simulink model "pmsm_hil"  (R2018b)
settings: Solver=VariableStepAuto  StartTime=0.0  StopTime=10.0  RelTol=1e-3
InitFcn:
  | pmsm_init;
values from neighbouring files (symbols this model uses):
  dt = 50e-9    (= 5e-08)    [pmsm_init.m]
  ImaxFX = 600    [pmsm_init.m]
  J = Tst*Tau/W    (= 0.15)    [pmsm_init.m]
  L = Ld    [pmsm_control_init.m]    (also in pmsm_init.m = [Ld Lq])
  pp = 3    [pmsm_init.m]
  Psi_PM = 66e-3    (= 0.066)    [pmsm_init.m]
  PsimaxFX = 2*abs(Psi_PM + Ld*Imax + j*Lq*Imax)    [pmsm_init.m]
  R = 18e-3    (= 0.018)    [pmsm_init.m]
  RPMmax = 60*1500/2/pi    (= 14323.9448783)    [pmsm_init.m]
  TaumaxFX = (3/2)*pp*real(j*(Psi_PM + Ld*Imax + j*Lq*Imax)*Imax*(-1+j))    [pmsm_init.m]
  Udc = 300    [pmsm_init.m]
  UmaxFX = 600    [pmsm_init.m]
  WmaxFX = 1500*pp    (= 4500)    [pmsm_init.m]
undefined symbols (not defined in the file or in its folder): j
libraries: simulink x2
settings Model: Creator=natlo  LastModifiedBy=Marci

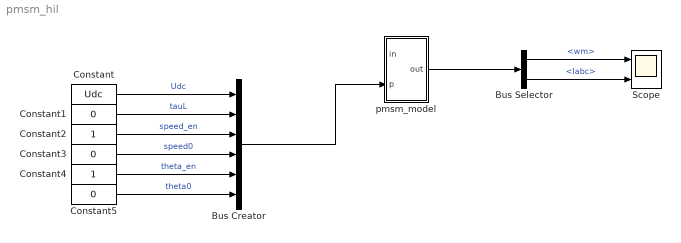
== system pmsm_hil ==
  Bus Creator : BusCreator  Inputs=6
  Bus Selector : BusSelector  OutputSignals=wm,Iabc
  Constant : Constant  Value=Udc  OutMax=[UmaxFX]  OutDataTypeStr=fixdt(1,vbits)  SampleTime=dt
  Constant1 : Constant  Value=0  OutMax=[TaumaxFX]  OutDataTypeStr=fixdt(1,vbits)  SampleTime=-1
  Constant2 : Constant  OutDataTypeStr=boolean  SampleTime=-1
  Constant3 : Constant  Value=0  OutMax=[RPMmax]  OutDataTypeStr=fixdt(1,vbits)  SampleTime=-1
  Constant4 : Constant  OutDataTypeStr=boolean  SampleTime=-1
  Constant5 : Constant  Value=0  OutMax=[180]  OutDataTypeStr=fixdt(1,vbits)  SampleTime=-1
  Scope : Scope  NumInputPorts=2
  pmsm_model : Subsystem
  wires:
  Constant5/1 -> Bus Creator/6  "theta0"
  Constant1/1 -> Bus Creator/2  "tauL"
  Constant2/1 -> Bus Creator/3  "speed_en"
  Constant/1 -> Bus Creator/1  "Udc"
  Constant3/1 -> Bus Creator/4  "speed0"
  Constant4/1 -> Bus Creator/5  "theta_en"
  Bus Creator/1 -> pmsm_model/2(p)
  pmsm_model/1(out) -> Bus Selector/1
  Bus Selector/1 -> Scope/1  "<wm>"
  Bus Selector/2 -> Scope/2  "<Iabc>"

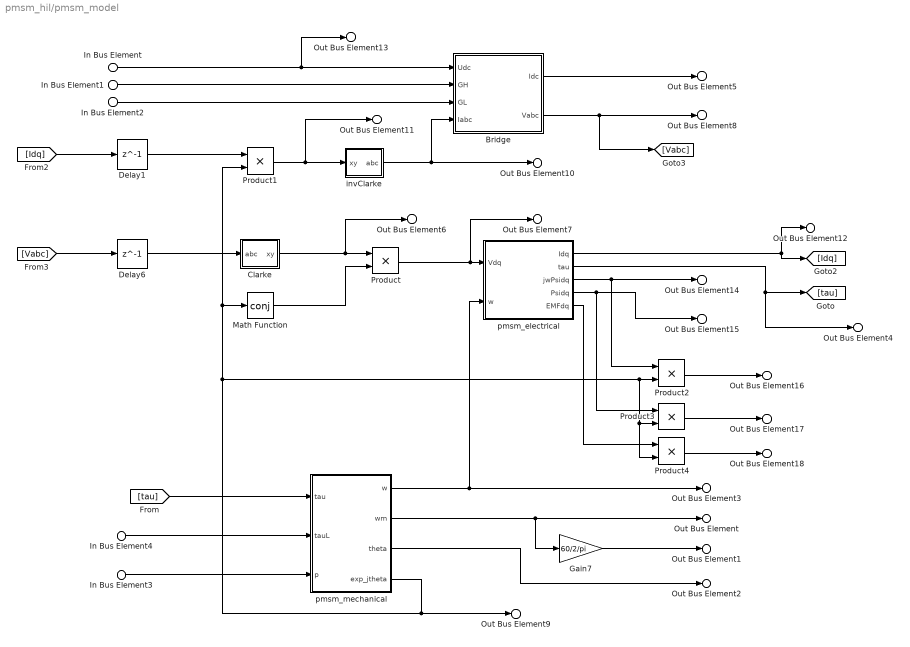
== system pmsm_hil/pmsm_model ==
  In Bus Element1 : Inport  PortName=in  Element=GH
  In Bus Element2 : Inport  PortName=in  Element=GL
  In Bus Element3 : Inport  Port=2  PortName=p
  In Bus Element : Inport  Port=2  PortName=p  Element=Udc
  In Bus Element4 : Inport  Port=2  PortName=p  Element=tauL
  Bridge : Subsystem
  Clarke : Subsystem
  Delay1 : Delay  DelayLength=1  InitialCondition=0
  Delay6 : Delay  DelayLength=1  InitialCondition=0
  Gain7 : Gain  Gain=60/2/pi  OutMax=[WmaxFX/pp*60/2/pi]  OutDataTypeStr=fixdt(1,vbits)
  Math Function : Math  Operator=conj  SaturateOnIntegerOverflow=on
  Product{,1..4} (5 alike) : Product  OutDataTypeStr=Inherit: Same as first input
  invClarke : Subsystem
  pmsm_electrical : Subsystem
  pmsm_mechanical : Subsystem
  Out Bus Element : Outport  PortName=out  Element=wm
  Out Bus Element1 : Outport  PortName=out  Element=rpm
  Out Bus Element2 : Outport  PortName=out  Element=theta
  Out Bus Element3 : Outport  PortName=out  Element=w
  Out Bus Element4 : Outport  PortName=out  Element=tau
  Out Bus Element5 : Outport  PortName=out  Element=Idc
  Out Bus Element6 : Outport  PortName=out  Element=Vxy
  Out Bus Element7 : Outport  PortName=out  Element=Vdq
  Out Bus Element8 : Outport  PortName=out  Element=Vabc
  Out Bus Element9 : Outport  PortName=out  Element=exp_jtheta
  Out Bus Element10 : Outport  PortName=out  Element=Iabc
  Out Bus Element11 : Outport  PortName=out  Element=Ixy
  Out Bus Element12 : Outport  PortName=out  Element=Idq
  Out Bus Element13 : Outport  PortName=out  Element=Udc
  Out Bus Element14 : Outport  PortName=out  Element=jwPsidq
  Out Bus Element15 : Outport  PortName=out  Element=Psidq
  Out Bus Element16 : Outport  PortName=out  Element=jwPsixy
  Out Bus Element17 : Outport  PortName=out  Element=Psixy
  Out Bus Element18 : Outport  PortName=out  Element=EMFxy
  wires:
  Product4/1 -> Out Bus Element18/1
  pmsm_electrical/5(EMFdq) -> Product4/1
  Product3/1 -> Out Bus Element17/1
  Product2/1 -> Out Bus Element16/1
  pmsm_electrical/4(Psidq) -> Product3/1, Out Bus Element15/1
  pmsm_electrical/3(jwPsidq) -> Out Bus Element14/1, Product2/1
  Delay6/1 -> Clarke/1(abc)
  Delay1/1 -> Product1/1
  In Bus Element/1 -> Bridge/1(Udc), Out Bus Element13/1
  In Bus Element1/1 -> Bridge/2(GH)
  In Bus Element2/1 -> Bridge/3(GL)
  Gain7/1 -> Out Bus Element1/1
  pmsm_mechanical/2(wm) -> Out Bus Element/1, Gain7/1
  pmsm_mechanical/3(theta) -> Out Bus Element2/1
  In Bus Element3/1 -> pmsm_mechanical/3(p)
  In Bus Element4/1 -> pmsm_mechanical/2(tauL)
  pmsm_electrical/2(tau) -> Out Bus Element4/1, [tau]
  [tau] -> pmsm_mechanical/1(tau)
  Bridge/1(Idc) -> Out Bus Element5/1
  Clarke/1(xy) -> Out Bus Element6/1, Product/1
  Math Function/1 -> Product/2
  Bridge/2(Vabc) -> Out Bus Element8/1, [Vabc]
  pmsm_mechanical/4(exp_jtheta) -> Product1/2, Math Function/1, Product2/2, Product3/2, Product4/2, Out Bus Element9/1
  [Idq] -> Delay1/1
  pmsm_electrical/1(Idq) -> Out Bus Element12/1, [Idq]
  Product/1 -> Out Bus Element7/1, pmsm_electrical/1(Vdq)
  pmsm_mechanical/1(w) -> Out Bus Element3/1, pmsm_electrical/2(w)
  [Vabc] -> Delay6/1
  Product1/1 -> invClarke/1(xy), Out Bus Element11/1
  invClarke/1(abc) -> Out Bus Element10/1, Bridge/4(Iabc)

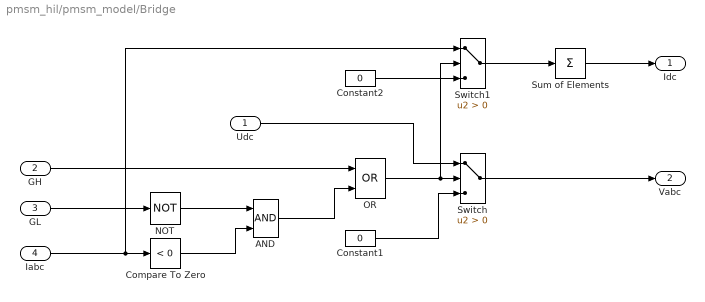
== system pmsm_hil/pmsm_model/Bridge ==
  Udc : Inport
  GH : Inport  Port=2
  GL : Inport  Port=3
  Iabc : Inport  Port=4
  AND : Logic  IconShape=distinctive  AllPortsSameDT=off  OutDataTypeStr=boolean
  Compare To Zero : simulink/Logic and Bit Operations/Compare To Zero  relop=<  OutDataTypeStr=boolean
  Constant1 : Constant  Value=0  OutDataTypeStr=Inherit: Inherit via back propagation  SampleTime=-1
  Constant2 : Constant  Value=0  OutDataTypeStr=Inherit: Inherit via back propagation  SampleTime=-1
  NOT : Logic  Operator=NOT  IconShape=distinctive  AllPortsSameDT=off  OutDataTypeStr=boolean
  OR : Logic  Operator=OR  IconShape=distinctive  AllPortsSameDT=off  OutDataTypeStr=boolean
  Sum of Elements : Sum  Inputs=+  OutMax=[ImaxFX]  OutDataTypeStr=fixdt(1,vbits)
  Switch : Switch  Criteria=u2 > Threshold
  Switch1 : Switch  Criteria=u2 > Threshold
  Idc : Outport
  Vabc : Outport  Port=2
  wires:
  Constant2/1 -> Switch1/3
  OR/1 -> Switch/2, Switch1/2
  Compare To Zero/1 -> AND/2
  Constant1/1 -> Switch/3
  GL/1 -> NOT/1
  Iabc/1 -> Switch1/1, Compare To Zero/1
  AND/1 -> OR/2
  Sum of Elements/1 -> Idc/1
  NOT/1 -> AND/1
  Switch1/1 -> Sum of Elements/1
  GH/1 -> OR/1
  Switch/1 -> Vabc/1
  Udc/1 -> Switch/1

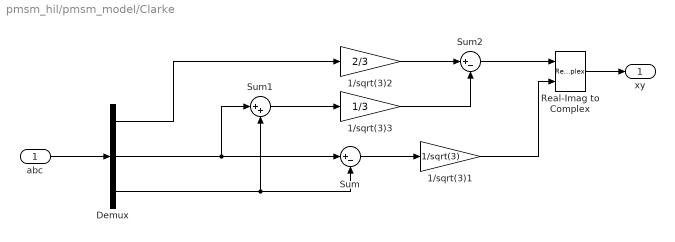
== system pmsm_hil/pmsm_model/Clarke ==
  abc : Inport
  1/sqrt(3)1 : Gain  Gain=1/sqrt(3)  ParamDataTypeStr=fixdt(1,cbits)  OutDataTypeStr=Inherit: Same as input
  1/sqrt(3)2 : Gain  Gain=2/3  ParamDataTypeStr=fixdt(1,cbits)  OutDataTypeStr=Inherit: Same as input
  1/sqrt(3)3 : Gain  Gain=1/3  ParamDataTypeStr=fixdt(1,cbits)  OutDataTypeStr=Inherit: Same as input
  Demux : Demux  Outputs=3
  Real-Imag to Complex : RealImagToComplex
  Sum : Sum  Inputs=|+-  OutDataTypeStr=Inherit: Same as accumulator
  Sum1 : Sum  Inputs=|++  OutDataTypeStr=Inherit: Same as accumulator
  Sum2 : Sum  Inputs=|+-  OutDataTypeStr=Inherit: Same as accumulator
  xy : Outport
  wires:
  Demux/3 -> Sum/2, Sum1/2
  1/sqrt(3)1/1 -> Real-Imag to Complex/2
  Demux/2 -> Sum/1, Sum1/1
  Sum/1 -> 1/sqrt(3)1/1
  1/sqrt(3)2/1 -> Sum2/1
  Sum1/1 -> 1/sqrt(3)3/1
  Demux/1 -> 1/sqrt(3)2/1
  Sum2/1 -> Real-Imag to Complex/1
  abc/1 -> Demux/1
  Real-Imag to Complex/1 -> xy/1
  1/sqrt(3)3/1 -> Sum2/2

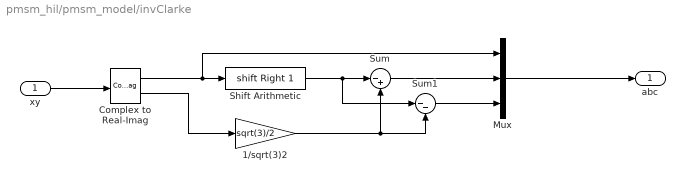
== system pmsm_hil/pmsm_model/invClarke ==
  xy : Inport
  1/sqrt(3)2 : Gain  Gain=sqrt(3)/2  ParamDataTypeStr=fixdt(1,cbits)  OutDataTypeStr=Inherit: Same as input
  Complex to Real-Imag : ComplexToRealImag
  Mux : Mux  Inputs=3
  Shift Arithmetic : ArithShift  BitShiftNumber=1  BitShiftDirection=Right
  Sum : Sum  Inputs=|-+  OutDataTypeStr=Inherit: Same as accumulator
  Sum1 : Sum  Inputs=|--  OutDataTypeStr=Inherit: Same as accumulator
  abc : Outport
  wires:
  xy/1 -> Complex to Real-Imag/1
  Mux/1 -> abc/1
  Complex to Real-Imag/2 -> 1/sqrt(3)2/1
  1/sqrt(3)2/1 -> Sum/2, Sum1/2
  Sum1/1 -> Mux/3
  Sum/1 -> Mux/2
  Shift Arithmetic/1 -> Sum1/1, Sum/1
  Complex to Real-Imag/1 -> Mux/1, Shift Arithmetic/1

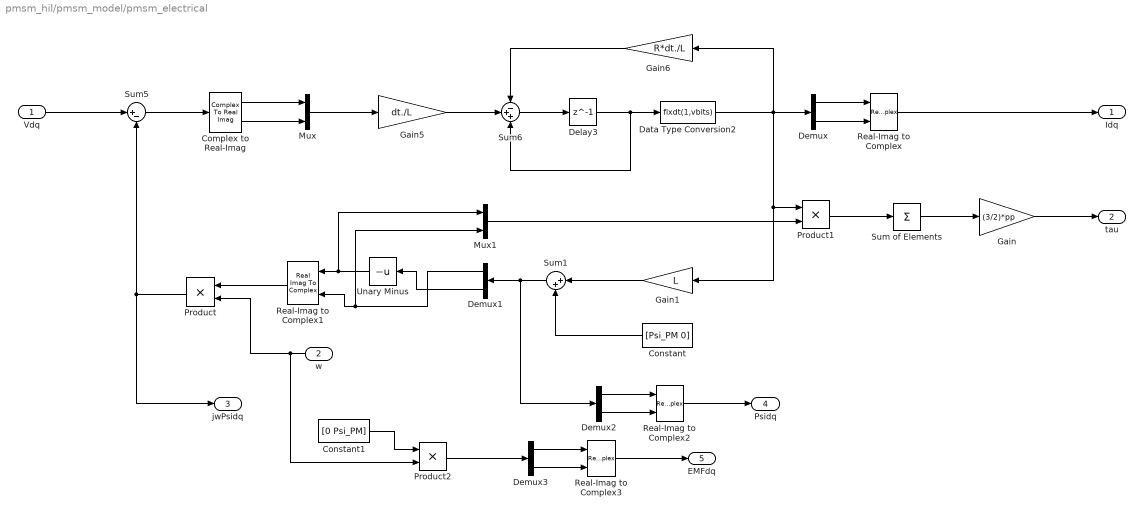
== system pmsm_hil/pmsm_model/pmsm_electrical ==
  Vdq : Inport
  w : Inport  Port=2
  Complex to Real-Imag : ComplexToRealImag
  Constant : Constant  Value=[Psi_PM 0]  OutDataTypeStr=fixdt(1,vbits)  SampleTime=-1
  Constant1 : Constant  Value=[0 Psi_PM]  OutDataTypeStr=fixdt(1,vbits)  SampleTime=-1
  Data Type Conversion2 : DataTypeConversion  OutMax=[ImaxFX]  OutDataTypeStr=fixdt(1,vbits)
  Delay3 : Delay  DelayLength=1  InitialCondition=0
  Demux{,1..3} (4 alike) : Demux  Outputs=2
  Gain : Gain  Gain=(3/2)*pp  ParamDataTypeStr=fixdt(1,cbits)  OutMax=[(3/2)*pp*PsimaxFX*ImaxFX]  OutDataTypeStr=fixdt(1,vbits)
  Gain1 : Gain  Gain=L  ParamDataTypeStr=fixdt(1,cbits)  OutMax=[max(L*ImaxFX)]  OutDataTypeStr=fixdt(1,vbits)
  Gain5 : Gain  Gain=dt./L  ParamDataTypeStr=fixdt(1,cbits)  OutMax=[max(dt./L*UmaxFX)]  OutDataTypeStr=fixdt(1,vbits)
  Gain6 : Gain  Gain=R*dt./L  ParamDataTypeStr=fixdt(1,cbits)  OutMax=[max(R*dt./L)*ImaxFX]  OutDataTypeStr=fixdt(1,vbits)
  Mux : Mux  Inputs=2
  Mux1 : Mux  Inputs=2
  Product : Product  OutMax=[UmaxFX]  OutDataTypeStr=fixdt(1,vbits)
  Product1 : Product  OutMax=[ImaxFX*PsimaxFX]  OutDataTypeStr=fixdt(1,vbits)
  Product2 : Product  OutMax=[UmaxFX]  OutDataTypeStr=fixdt(1,vbits)
  Real-Imag to Complex{,1..3} (4 alike) : RealImagToComplex
  Sum of Elements : Sum  Inputs=+  OutDataTypeStr=Inherit: Same as accumulator
  Sum1 : Sum  Inputs=|++  OutDataTypeStr=Inherit: Same as accumulator
  Sum5 : Sum  Inputs=|+-  OutDataTypeStr=Inherit: Same as accumulator
  Sum6 : Sum  Inputs=-++  OutDataTypeStr=fixdt(1,44,33)
  Unary Minus : UnaryMinus
  Idq : Outport
  tau : Outport  Port=2
  jwPsidq : Outport  Port=3
  Psidq : Outport  Port=4
  EMFdq : Outport  Port=5
  wires:
  Constant1/1 -> Product2/1
  Real-Imag to Complex3/1 -> EMFdq/1
  Product2/1 -> Demux3/1
  Demux3/1 -> Real-Imag to Complex3/1
  Demux3/2 -> Real-Imag to Complex3/2
  Real-Imag to Complex2/1 -> Psidq/1
  Demux2/2 -> Real-Imag to Complex2/2
  Demux2/1 -> Real-Imag to Complex2/1
  Sum1/1 -> Demux1/1, Demux2/1
  Gain5/1 -> Sum6/2
  Sum6/1 -> Delay3/1
  Gain/1 -> tau/1
  Mux/1 -> Gain5/1
  Data Type Conversion2/1 -> Product1/1, Gain1/1, Demux/1, Gain6/1
  Demux1/2 -> Unary Minus/1
  Demux/1 -> Real-Imag to Complex/1
  Delay3/1 -> Data Type Conversion2/1, Sum6/3
  Demux/2 -> Real-Imag to Complex/2
  Constant/1 -> Sum1/2
  Demux1/1 -> Mux1/2, Real-Imag to Complex1/2
  Product1/1 -> Sum of Elements/1
  Gain1/1 -> Sum1/1
  Product/1 -> Sum5/2, jwPsidq/1
  Gain6/1 -> Sum6/1
  Unary Minus/1 -> Mux1/1, Real-Imag to Complex1/1
  Complex to Real-Imag/1 -> Mux/1
  w/1 -> Product/2, Product2/2
  Vdq/1 -> Sum5/1
  Complex to Real-Imag/2 -> Mux/2
  Sum5/1 -> Complex to Real-Imag/1
  Mux1/1 -> Product1/2
  Sum of Elements/1 -> Gain/1
  Real-Imag to Complex1/1 -> Product/1
  Real-Imag to Complex/1 -> Idq/1

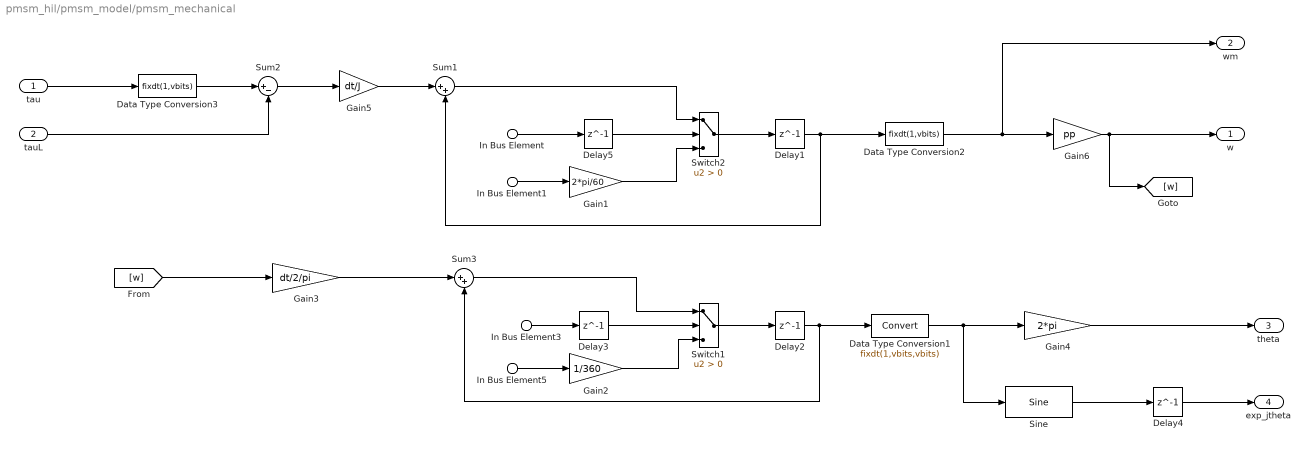
== system pmsm_hil/pmsm_model/pmsm_mechanical ==
  tau : Inport
  tauL : Inport  Port=2
  In Bus Element : Inport  Port=3  PortName=p  Element=speed_en
  In Bus Element1 : Inport  Port=3  PortName=p  Element=speed0
  In Bus Element3 : Inport  Port=3  PortName=p  Element=theta_en
  In Bus Element5 : Inport  Port=3  PortName=p  Element=theta0
  Data Type Conversion1 : DataTypeConversion  OutDataTypeStr=fixdt(1,vbits,vbits)
  Data Type Conversion2 : DataTypeConversion  OutMax=[WmaxFX/pp]  OutDataTypeStr=fixdt(1,vbits)
  Data Type Conversion3 : DataTypeConversion  OutMax=[TaumaxFX]  OutDataTypeStr=fixdt(1,vbits)
  Delay{1..5} (5 alike) : Delay  DelayLength=1  InitialCondition=0
  Gain1 : Gain  Gain=2*pi/60  ParamDataTypeStr=fixdt(1,cbits)  OutMax=[WmaxFX/pp]  OutDataTypeStr=fixdt(1,vbits)
  Gain2 : Gain  Gain=1/360  OutMax=[0.5]  OutDataTypeStr=fixdt(1,vbits)
  Gain3 : Gain  Gain=dt/2/pi  ParamDataTypeStr=fixdt(1,cbits)  OutMax=[WmaxFX*dt/2/pi]  OutDataTypeStr=fixdt(1,vbits)
  Gain4 : Gain  Gain=2*pi  ParamDataTypeStr=fixdt(1,cbits)  OutMax=[pi]  OutDataTypeStr=fixdt(1,vbits)
  Gain5 : Gain  Gain=dt/J  ParamDataTypeStr=fixdt(1,cbits)  OutMax=[dt/J*TaumaxFX]  OutDataTypeStr=fixdt(1,vbits)
  Gain6 : Gain  Gain=pp  OutMax=[WmaxFX]  OutDataTypeStr=fixdt(1,vbits)
  Sine : simulink/Lookup Tables/Sine  Formula=exp(j*2*pi*u)  NumDataPoints=(2^5)+1  OutputWordLength=16  InternalRulePriority=Speed
      settings: SourceProductName=Simulink
  Sum1 : Sum  Inputs=|++  OutDataTypeStr=fixdt(1,12+37,37)
  Sum2 : Sum  Inputs=|+-  OutDataTypeStr=Inherit: Same as accumulator
  Sum3 : Sum  Inputs=|++  OutDataTypeStr=fixdt(1,38,38)
  Switch1 : Switch  Criteria=u2 > Threshold
  Switch2 : Switch  Criteria=u2 > Threshold
  w : Outport
  wm : Outport  Port=2
  theta : Outport  Port=3
  exp_jtheta : Outport  Port=4
  wires:
  Delay4/1 -> exp_jtheta/1
  Sine/1 -> Delay4/1
  Sum2/1 -> Gain5/1
  Delay1/1 -> Data Type Conversion2/1, Sum1/2
  tauL/1 -> Sum2/2
  Gain6/1 -> w/1, [w]
  tau/1 -> Data Type Conversion3/1
  Sum1/1 -> Switch2/1
  Gain5/1 -> Sum1/1
  Delay5/1 -> Switch2/2
  Switch2/1 -> Delay1/1
  In Bus Element1/1 -> Gain1/1
  In Bus Element/1 -> Delay5/1
  Gain1/1 -> Switch2/3
  Gain3/1 -> Sum3/1
  Delay2/1 -> Data Type Conversion1/1, Sum3/2
  Sum3/1 -> Switch1/1
  Delay3/1 -> Switch1/2
  Gain2/1 -> Switch1/3
  Switch1/1 -> Delay2/1
  In Bus Element3/1 -> Delay3/1
  In Bus Element5/1 -> Gain2/1
  [w] -> Gain3/1
  Data Type Conversion2/1 -> wm/1, Gain6/1
  Data Type Conversion1/1 -> Sine/1, Gain4/1
  Data Type Conversion3/1 -> Sum2/1
  Gain4/1 -> theta/1
